simulink model "sensorRPM"  (R2023a)
settings: Solver=VariableStepAuto  StartTime=0.0  StopTime=10.0  RelTol=1e-3
settings Model: Creator=rafael  LastModifiedBy=rafael

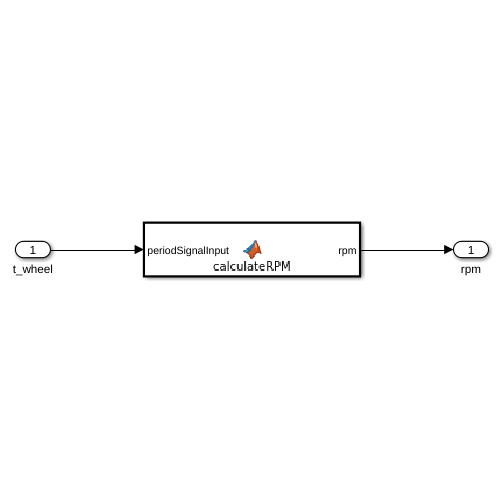
[thumbnail: Simulink's stored preview of the top-level diagram]
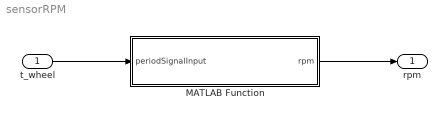
== system sensorRPM ==
  t_wheel : Inport
  MATLAB Function : MATLAB Function  TreatAsAtomicUnit=on
  rpm : Outport
  wires:
  t_wheel/1 -> MATLAB Function/1(periodSignalInput)
  MATLAB Function/1(rpm) -> rpm/1

== matlab function sensorRPM/MATLAB Function ==
  data: periodSignalInput input; rpm output
function rpm = calculateRPM(periodSignalInput)
    % FUNCTION Calculate Air Tempperature [K]
    rpm = 1e6 / (periodSignalInput * 128);
end
